simulink model "simu_control_robot_5"  (Simulink 7.9)
settings: Solver=ode3  StartTime=0  StopTime=1.190000e+00  FixedStep=1.000000e-02  RelTol=1e-3
values from neighbouring files (symbols this model uses):
  xsx_d = repmat(0,duration_disc,1)    [WPG_results_10.m]    (also in WPG_results_2.m = zmp.A_xcom_spd(1:sum(wpg_param.discretization(1:wpg_param.nb; WPG_results_3.m = zmp.A_xcom_spd(1:sum(wpg_param.discretization(1:wpg_param.nb; WPG_results_4.m = repmat(zmp.A_xcom_spd(1,:)*wpg_param.psa_abcdDSP(1:size(zmp.; WPG_results_5.m = [time xsx_d-xsx_d_init])
  xx_d = repmat(trajectories_zmp.xpcom(1),duration_disc,1)    [WPG_results_10.m]    (also in WPG_results_2.m = trajectories_zmp.xpcom(1:sum(wpg_param.discretization(1:wpg_; WPG_results_3.m = trajectories_zmp.xpcom(1:sum(wpg_param.discretization(1:wpg_; WPG_results_4.m; WPG_results_5.m = [time xx_d-xx_d_init])
  ysx_d = repmat(0,duration_disc,1)    [WPG_results_10.m]    (also in WPG_results_2.m = zmp.A_ycom_spd(1:sum(wpg_param.discretization(1:wpg_param.nb; WPG_results_3.m = zmp.A_ycom_spd(1:sum(wpg_param.discretization(1:wpg_param.nb; WPG_results_4.m = repmat(zmp.A_ycom_spd(1,:)*wpg_param.psa_abcdDSP(end/2+1:end; WPG_results_5.m = [time ysx_d-ysx_d_init])
  yx_d = repmat(0,duration_disc,1)    [WPG_results_10.m]    (also in WPG_results_2.m = trajectories_zmp.ypcom(1:sum(wpg_param.discretization(1:wpg_; WPG_results_3.m = trajectories_zmp.ypcom(1:sum(wpg_param.discretization(1:wpg_; WPG_results_4.m = repmat(trajectories_zmp.ypcom(1),duration_disc,1); WPG_results_5.m = [time yx_d-yx_d_init])
settings Model: Creator=pajon  LastModifiedBy=pajon

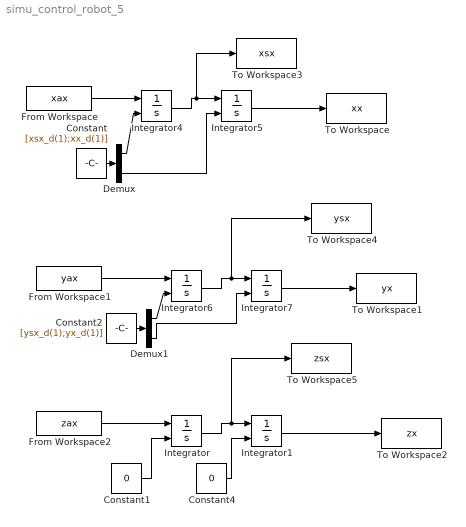
== system simu_control_robot_5 ==
  Constant : Constant  Value=[xsx_d(1);xx_d(1)]
  Constant1 : Constant  Value=0
  Constant2 : Constant  Value=[ysx_d(1);yx_d(1)]
  Constant4 : Constant  Value=0
  Demux : Demux  Outputs=2
  Demux1 : Demux  Outputs=2
  From Workspace : FromWorkspace  VariableName=xax  SampleTime=0
  From Workspace1 : FromWorkspace  VariableName=yax  SampleTime=0
  From Workspace2 : FromWorkspace  VariableName=zax  SampleTime=0
  Integrator : Integrator  InitialConditionSource=external  InitialCondition=xsx_d(1,2)
  Integrator1 : Integrator  InitialConditionSource=external  InitialCondition=xx_d(1,2)
  Integrator4 : Integrator  InitialConditionSource=external  InitialCondition=xsx_d(1,2)
  Integrator5 : Integrator  InitialConditionSource=external  InitialCondition=xx_d(1,2)
  Integrator6 : Integrator  InitialConditionSource=external  InitialCondition=xsx_d(1,2)
  Integrator7 : Integrator  InitialConditionSource=external  InitialCondition=xx_d(1,2)
  To Workspace : ToWorkspace  VariableName=xx  SampleTime=-1  SaveFormat=Timeseries
  To Workspace1 : ToWorkspace  VariableName=yx  SampleTime=-1  SaveFormat=Timeseries
  To Workspace2 : ToWorkspace  VariableName=zx  SampleTime=-1  SaveFormat=Timeseries
  To Workspace3 : ToWorkspace  VariableName=xsx  SampleTime=-1  SaveFormat=Timeseries
  To Workspace4 : ToWorkspace  VariableName=ysx  SampleTime=-1  SaveFormat=Timeseries
  To Workspace5 : ToWorkspace  VariableName=zsx  SampleTime=-1  SaveFormat=Timeseries
  wires:
  Constant2/1 -> Demux1/1
  Constant/1 -> Demux/1
  Integrator/1 -> Integrator1/1, To Workspace5/1
  Constant1/1 -> Integrator/2
  Constant4/1 -> Integrator1/2
  Integrator4/1 -> Integrator5/1, To Workspace3/1
  Integrator6/1 -> Integrator7/1, To Workspace4/1
  Demux/1 -> Integrator4/2
  Demux/2 -> Integrator5/2
  Demux1/1 -> Integrator6/2
  Demux1/2 -> Integrator7/2
  From Workspace2/1 -> Integrator/1
  From Workspace1/1 -> Integrator6/1
  Integrator5/1 -> To Workspace/1
  Integrator7/1 -> To Workspace1/1
  Integrator1/1 -> To Workspace2/1
  From Workspace/1 -> Integrator4/1
